simulink model "mcb_pmsm_foc_sensorless_CVAC_IF_f28379d"  (R2026a)
settings: Solver=FixedStepDiscrete  StopTime=8  EnableMultiTasking=on
InitFcn:
  | cvac_if_model_init;
model workspace (MAT data in the model file):
  encoderResolution = 2000
  hallOffset = '0.5'
  indexOffset = 850
  polePairs = '4'
values from neighbouring files (symbols this model uses):
  acceleration = 500 / PU_System.N_base    [cvac_if_model_init.m]
  CVAC_IF_Mode = uint8(2)    [cvac_if_model_init.m]
  CVAC_LoadConstant = CVAC_LoadFinal    [cvac_if_model_init.m]
  PU_System = mcb.getPUSystemParameters(pmsm, inverter)    [cvac_if_model_init.m]
  Speed_openLoop_PU = 400 / PU_System.N_base    [cvac_if_model_init.m]
  Ts = single(param.TsFast)    [cvac_if_reference_fast_step.m]
undefined symbols (not defined in the file or in its folder): bit, CVAC_LoadFinal, CVAC_LoadInitial, CVAC_LoadStepTime, dataType, Down, GPTRIP1SEL, GPTRIP2SEL, inverter, NumBits1, NumBits2, PI_params, pmsm, Slope1, Slope2, target, Ts_motor, Ts_simulink, Ts_speed, TZ1, TZ2, Up
libraries: mcbcontrolslib x9, c2802xlib x7, simulink x6, c280xlib x5, mcbeeMathTransformLib x4, c2837xDlib x4, mcbpositiondecoderlib x3, slpidlib x3, sl_signal_attributes x2, mcbpmsmiflib x2, mcbsensorlessestimatorlib x1, svdschedulerlib x1
(part 3 of 3)

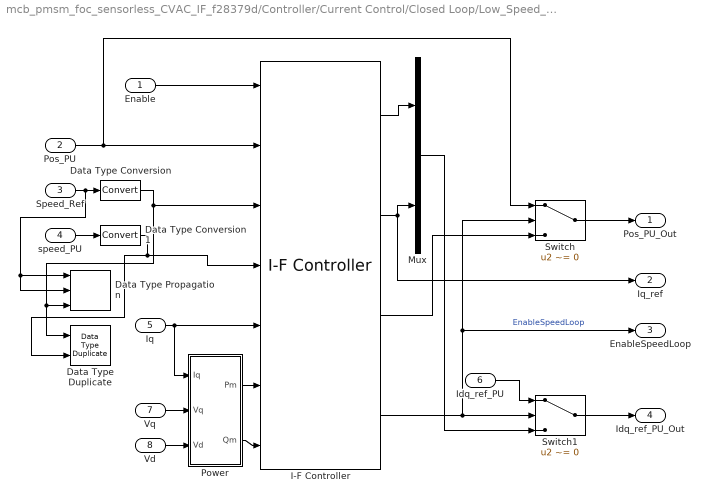
== system mcb_pmsm_foc_sensorless_CVAC_IF_f28379d/Controller/Current Control/Closed Loop/Low_Speed_Control/Variant Subsystem/WithPowerOptimzation ==
  Enable : Inport
  Pos_PU : Inport  Port=2
  Speed_Ref : Inport  Port=3
  speed_PU : Inport  Port=4
  Iq : Inport  Port=5
  Idq_ref_PU : Inport  Port=6
  Vq : Inport  Port=7
  Vd : Inport  Port=8
  Data Type Duplicate : DataTypeDuplicate
  Data Type Propagation : sl_signal_attributes/Data Type Propagation  PropDataType=fixdt(1, 16)  IfRefDouble=double  IfRefSingle=single  IsSigned=IsSigned1 or IsSigned2  NumBitsBase=max([NumBits1 NumBits2])  NumBitsMult=1  NumBitsAdd=0  NumBitsAllowFinal=-1  PropScalingMode=Obtain via best precision  PropScaling=2^-10  ValuesUsedBestPrec=[4 -4]  SlopeBase=min([Slope1 Slope2])  SlopeMult=1  SlopeAdd=0  BiasBase=Bias1  BiasMult=1  BiasAdd=0
      settings: LibrarySourceBlock=|
      | simulink/Signal
      | Attributes/Data Type
      | Propagation
  Data Type Conversion : DataTypeConversion  SaturateOnIntegerOverflow=off  RndMeth=Floor
  Data Type Conversion1 : DataTypeConversion  SaturateOnIntegerOverflow=off  RndMeth=Floor
  I-F Controller : mcbpmsmiflib/I-F Controller  EnableSpeedDamp=on  ParameterBusInput=off  PolePairs=pmsm.p  PositionUnit=Per-unit  SpeedUnit=Per-unit  PerUnitSpeed=PU_System.N_base  CurrentUnit=Per-unit  TempCurrentUnit=Per-unit  MaxStatorCurrent=PU_System.I_base  BlkSampleTime=Ts  CurrentLimitObjective=Reduce power consumption (Optimize load current)  OlClSpeed=PU_System.N_base*Speed_openLoop_PU  ClOlSpeed=PU_System.N_base*Speed_openLoop_PU*0.5  MaxStartingCurrent=pmsm.I_rated  MaxAcceleration=0.1*pmsm.T_rated/pmsm.J  CurrentDownSlope=10*pmsm.I_rated  IdleTime=1  Angle=(10/360)*2*pi  VoltageUnit=Per-unit  TempVoltageUnit=Per-unit  MaxStatorVoltage=PU_System.V_base  DampCoeff=2.6172/(PU_System.N_base*Speed_openLoop_PU)  PowerUnit=SI unit  TempPowerUnit=SI unit  MaxInpPower=100  PwrFactor=1.5  Kp=1e-4*PU_System.I_base  Ki=1e-1*PU_System.I_base
  Mux : Mux  Inputs=2
  Power : Subsystem
  Switch : Switch  Criteria=u2 ~= 0  Threshold=0.1  SaturateOnIntegerOverflow=off  InputSameDT=off  OutDataTypeStr=Inherit: Same as first input
  Switch1 : Switch  Criteria=u2 ~= 0  Threshold=0.1  SaturateOnIntegerOverflow=off  InputSameDT=off  OutDataTypeStr=Inherit: Same as first input
  Pos_PU_Out : Outport
  Iq_ref : Outport  Port=2
  EnableSpeedLoop : Outport  Port=3
  Idq_ref_PU_Out : Outport  Port=4
  wires:
  Switch/1 -> Pos_PU_Out/1
  I-F Controller/3 -> Switch/3
  Data Type Conversion/1 -> Data Type Duplicate/1, Data Type Propagation/3, I-F Controller/3
  Pos_PU/1 -> I-F Controller/2, Switch/1
  Speed_Ref/1 -> Data Type Propagation/2, Data Type Propagation/1, Data Type Conversion/1
  Data Type Conversion1/1 -> Data Type Duplicate/2, I-F Controller/4
  Enable/1 -> I-F Controller/1
  Mux/1 -> Switch1/3
  speed_PU/1 -> Data Type Conversion1/1
  I-F Controller/1 -> Mux/1
  I-F Controller/4 -> EnableSpeedLoop/1, Switch/2, Switch1/2  "EnableSpeedLoop"
  Iq/1 -> Power/1(Iq), I-F Controller/5
  I-F Controller/2 -> Mux/2, Iq_ref/1
  Switch1/1 -> Idq_ref_PU_Out/1
  Idq_ref_PU/1 -> Switch1/1
  Power/2(Qm) -> I-F Controller/7
  Vq/1 -> Power/2(Vq)
  Vd/1 -> Power/3(Vd)
  Power/1(Pm) -> I-F Controller/6

== system mcb_pmsm_foc_sensorless_CVAC_IF_f28379d/Controller/Hardware Init/Variant Subsystem/Code Generation/Calculate ADC Offset /For Iterator Subsystem ==
  ADC_B2 : c2802xlib/ADC  Priority=20  blkParamProc=C2000_Type4  ADCModule=B  samplingMode=Single sample mode  ADCResolution=12-bit (Single-ended input)  ADC29xResolution=12-bit  ADCMode=Single-ended input  useSOC1=SOC2  useSOC2=SOC0_SOC1  SOCAcquisitionWindow=15  SOCTriggerSource=Software  SOCInterruptTrigger=No ADCINT  Ts=-1  dType=uint16  postInterrupt=off  interruptSel=ADCINT1  ADCINTContinuous=on  endma=off  chdma=1  conv1=ADCINA0  conv2=ADCINA0 and ADCINB0  conv1_Type4=ADCIN2  conv2_Type4=ADCIN0 and ADCIN1
  ADC_C2 : c2802xlib/ADC  Priority=20  blkParamProc=C2000_Type4  ADCModule=C  samplingMode=Single sample mode  ADCResolution=12-bit (Single-ended input)  ADC29xResolution=12-bit  ADCMode=Single-ended input  useSOC1=SOC2  useSOC2=SOC0_SOC1  SOCAcquisitionWindow=15  SOCTriggerSource=Software  SOCInterruptTrigger=No ADCINT  Ts=-1  dType=uint16  postInterrupt=off  interruptSel=ADCINT1  ADCINTContinuous=on  endma=off  chdma=1  conv1=ADCINA0  conv2=ADCINA0 and ADCINB0  conv1_Type4=ADCIN2  conv2_Type4=ADCIN0 and ADCIN1
  For Iterator : ForIterator  IterationLimit=16  IterationVariableDataType=uint16
  If : If  IfExpression=u1 > 8  ShowElse=off
  If Action Subsystem : Subsystem  TreatAsAtomicUnit=on
  Out1 : Outport
  Out2 : Outport  Port=2
  wires:
  For Iterator/1 -> If/1
  ADC_C2/1 -> If Action Subsystem/1(In1)
  ADC_B2/1 -> If Action Subsystem/2(In2)
  If Action Subsystem/1(Out1) -> Out1/1
  If Action Subsystem/2(Out2) -> Out2/1
  If/1 -> If Action Subsystem/Action

== system mcb_pmsm_foc_sensorless_CVAC_IF_f28379d/Controller/Hardware Init/Variant Subsystem/Code Generation/Calculate ADC Offset /If Action Subsystem ==
  In1 : Inport
  Action Port : ActionPort  ActionPortLabel=if(u1 > u3 & u1 < u2)
  Data Store Write1 : DataStoreWrite  DataStoreName=IaOffset  IndexOptions=Index vector (dialog)  Indices=1  OutputSizes=1
  wires:
  In1/1 -> Data Store Write1/1

== system mcb_pmsm_foc_sensorless_CVAC_IF_f28379d/Controller/Hardware Init/Variant Subsystem/Code Generation/Calculate ADC Offset /If Action Subsystem1 ==
  Action Port : ActionPort  ActionPortLabel=else
  Constant : Constant  Value=inverter.CtSensAOffset  OutDataTypeStr=Inherit: Inherit via back propagation
  Data Store Write1 : DataStoreWrite  DataStoreName=IaOffset  IndexOptions=Index vector (dialog)  Indices=1  OutputSizes=1
  wires:
  Constant/1 -> Data Store Write1/1

== system mcb_pmsm_foc_sensorless_CVAC_IF_f28379d/Controller/Hardware Init/Variant Subsystem/Code Generation/Calculate ADC Offset /If Action Subsystem2 ==
  In1 : Inport
  Action Port : ActionPort  ActionPortLabel=if(u1 > u3 & u1 < u2)
  Data Store Write2 : DataStoreWrite  DataStoreName=IbOffset  IndexOptions=Index vector (dialog)  Indices=1  OutputSizes=1
  wires:
  In1/1 -> Data Store Write2/1

== system mcb_pmsm_foc_sensorless_CVAC_IF_f28379d/Controller/Hardware Init/Variant Subsystem/Code Generation/Calculate ADC Offset /If Action Subsystem3 ==
  Action Port : ActionPort  ActionPortLabel=else
  Constant1 : Constant  Value=inverter.CtSensBOffset  OutDataTypeStr=Inherit: Inherit via back propagation
  Data Store Write2 : DataStoreWrite  DataStoreName=IbOffset  IndexOptions=Index vector (dialog)  Indices=1  OutputSizes=1
  wires:
  Constant1/1 -> Data Store Write2/1

== system mcb_pmsm_foc_sensorless_CVAC_IF_f28379d/Controller/Hardware Init/Variant Subsystem/Code Generation/DRV Enable/ADC Gain Setting ==
  In1 : Inport
  Enable : EnablePort
  Demux : Demux  Outputs=2
  Display : Display
      settings: Format=hex (Stored Integer)
  Display1 : Display
      settings: Format=hex (Stored Integer)
  SPI Master Transfer : c280xlib/SPI Controller Transfer  SPISelect=SPI_A  ClockPolarity=Rising_edge  ClockPhase=No_delay  SPIModule=uint32(0)  Mode=Master  BusSpeed=uint32(1000000)  FirstBitToTransfer=Most significant bit (MSB)  ClockMode=0  BlockFunction=Transfer  EnableRegisterAddress=off  RegisterAddress=0  OutputDataType=int8  OutputDataLength=1  DataBits=16  UseCustomSSPin=Provided by the SPI peripheral  ActiveLowSSPin=Active low  Pin=61
  SPI Master Transfer1 : c280xlib/SPI Controller Transfer  SPISelect=SPI_A  ClockPolarity=Rising_edge  ClockPhase=No_delay  SPIModule=uint32(0)  Mode=Master  BusSpeed=uint32(1000000)  FirstBitToTransfer=Most significant bit (MSB)  ClockMode=0  BlockFunction=Transfer  EnableRegisterAddress=off  RegisterAddress=0  OutputDataType=int8  OutputDataLength=1  DataBits=16  UseCustomSSPin=Provided by the SPI peripheral  ActiveLowSSPin=Active low  Pin=61
  wires:
  Demux/2 -> SPI Master Transfer1/1
  SPI Master Transfer/1 -> Display/1
  SPI Master Transfer1/1 -> Display1/1
  Demux/1 -> SPI Master Transfer/1
  In1/1 -> Demux/1

== system mcb_pmsm_foc_sensorless_CVAC_IF_f28379d/Controller/Serial Receive/SCI_Rx/Simulation/Data_Conditioning_Tx/Data_Type_Fixed_Point ==
  In1 : Inport
  In2 : Inport  Port=2
  Data Type Conversion : DataTypeConversion  OutDataTypeStr=fixdt(1,32,28)  RndMeth=Simplest  SaturateOnIntegerOverflow=off
  Data Type Conversion1 : DataTypeConversion  OutDataTypeStr=uint32  RndMeth=Simplest  SaturateOnIntegerOverflow=off
  Data Type Conversion3 : DataTypeConversion  OutDataTypeStr=uint32  ConvertRealWorld=Stored Integer (SI)  RndMeth=Simplest  SaturateOnIntegerOverflow=off
  Mux : Mux  Inputs=2
  Data : Outport
  wires:
  In1/1 -> Data Type Conversion/1
  Data Type Conversion3/1 -> Mux/1
  Data Type Conversion/1 -> Data Type Conversion3/1
  In2/1 -> Data Type Conversion1/1
  Data Type Conversion1/1 -> Mux/2
  Mux/1 -> Data/1

== system mcb_pmsm_foc_sensorless_CVAC_IF_f28379d/Controller/Serial Receive/SCI_Rx/Simulation/Data_Conditioning_Tx/Data_Type_Float ==
  In1 : Inport
  In2 : Inport  Port=2
  Data Type Conversion2 : DataTypeConversion  OutDataTypeStr=single  RndMeth=Simplest  SaturateOnIntegerOverflow=off
  Mux : Mux  Inputs=2
  Data : Outport
  wires:
  In1/1 -> Mux/1
  Mux/1 -> Data/1
  In2/1 -> Data Type Conversion2/1
  Data Type Conversion2/1 -> Mux/2

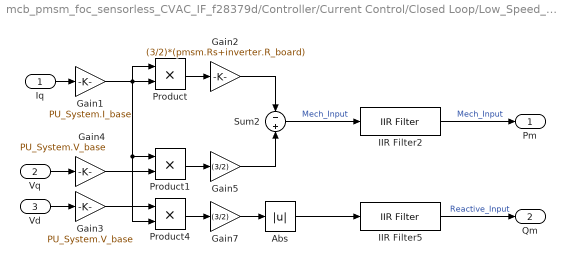
== system mcb_pmsm_foc_sensorless_CVAC_IF_f28379d/Controller/Current Control/Closed Loop/Low_Speed_Control/Variant Subsystem/WithPowerOptimzation/Power ==
  Iq : Inport
  Vq : Inport  Port=2
  Vd : Inport  Port=3
  Abs : Abs  SaturateOnIntegerOverflow=off
  Gain1 : Gain  Gain=PU_System.I_base  OutDataTypeStr=Inherit: Inherit via back propagation  RndMeth=Simplest
  Gain2 : Gain  Gain=(3/2)*(pmsm.Rs+inverter.R_board)  OutDataTypeStr=Inherit: Inherit via back propagation  RndMeth=Simplest
  Gain3 : Gain  Gain=PU_System.V_base  OutDataTypeStr=Inherit: Inherit via back propagation  RndMeth=Simplest
  Gain4 : Gain  Gain=PU_System.V_base  OutDataTypeStr=Inherit: Inherit via back propagation  RndMeth=Simplest
  Gain5 : Gain  Gain=(3/2)  OutDataTypeStr=Inherit: Inherit via back propagation  RndMeth=Simplest
  Gain7 : Gain  Gain=(3/2)  OutDataTypeStr=Inherit: Inherit via back propagation  RndMeth=Simplest
  IIR Filter2 : mcbcontrolslib/IIR Filter  VariantControl=Low Pass Filter  VariantSelect=Low-pass  FilterConstantInputType=Specify via dialog  Filter_constant=0.001  InitialOutput=Specify via dialog  InitialOutputValue=0  ExternalReset=none  advancedSettings=on  Ts=50e-6  cutOff_freq=3.1863
      settings: LibrarySourceBlock=mcblib/Signal Management/IIR Filter
  IIR Filter5 : mcbcontrolslib/IIR Filter  VariantControl=Low Pass Filter  VariantSelect=Low-pass  FilterConstantInputType=Specify via dialog  Filter_constant=0.001  InitialOutput=Specify via dialog  InitialOutputValue=0  ExternalReset=none  advancedSettings=on  Ts=50e-6  cutOff_freq=3.1863
      settings: LibrarySourceBlock=mcblib/Signal Management/IIR Filter
  Product : Product  OutDataTypeStr=Inherit: Inherit via back propagation  RndMeth=Simplest
  Product1 : Product  OutDataTypeStr=Inherit: Inherit via back propagation  RndMeth=Simplest
  Product4 : Product  OutDataTypeStr=Inherit: Inherit via back propagation  RndMeth=Simplest
  Sum2 : Sum  Inputs=-+
  Pm : Outport
  Qm : Outport  Port=2
  wires:
  Sum2/1 -> IIR Filter2/1  "Mech_Input"
  Product4/1 -> Gain7/1
  IIR Filter5/1 -> Qm/1  "Reactive_Input"
  Gain5/1 -> Sum2/2
  Gain7/1 -> Abs/1
  Iq/1 -> Gain1/1
  Gain3/1 -> Product4/1
  Vq/1 -> Gain4/1
  Gain4/1 -> Product1/2
  Abs/1 -> IIR Filter5/1
  Product/1 -> Gain2/1
  Product1/1 -> Gain5/1
  IIR Filter2/1 -> Pm/1  "Mech_Input"
  Gain1/1 -> Product4/2, Product1/1, Product/1, Product/2
  Vd/1 -> Gain3/1
  Gain2/1 -> Sum2/1

== system mcb_pmsm_foc_sensorless_CVAC_IF_f28379d/Controller/Hardware Init/Variant Subsystem/Code Generation/Calculate ADC Offset /For Iterator Subsystem/If Action Subsystem ==
  In1 : Inport
  In2 : Inport  Port=2
  Action Port : ActionPort  ActionPortLabel=if(u1 > 8)
  Memory : Memory  InheritSampleTime=on
  Memory1 : Memory  InheritSampleTime=on
  Sum : Sum
  Sum1 : Sum
  Out1 : Outport
  Out2 : Outport  Port=2
  wires:
  In1/1 -> Sum/1
  Sum/1 -> Out1/1, Memory/1
  In2/1 -> Sum1/1
  Memory/1 -> Sum/2
  Sum1/1 -> Out2/1, Memory1/1
  Memory1/1 -> Sum1/2
